simulink model "feedback_system"  (R2015a)
settings: Solver=ode45  StartTime=0.0  StopTime=t_stop  MaxStep=1e-4  MinStep=1e-5  RelTol=1e-3
undefined symbols (not defined in the file): delta_a, delta_y, rho, wy
libraries: cstblocks x2, simulink x1
settings Model: Creator=Berk Delibalta  LastModifiedBy=Berk Delibalta
settings SolverCC: InitialStep=1e-5

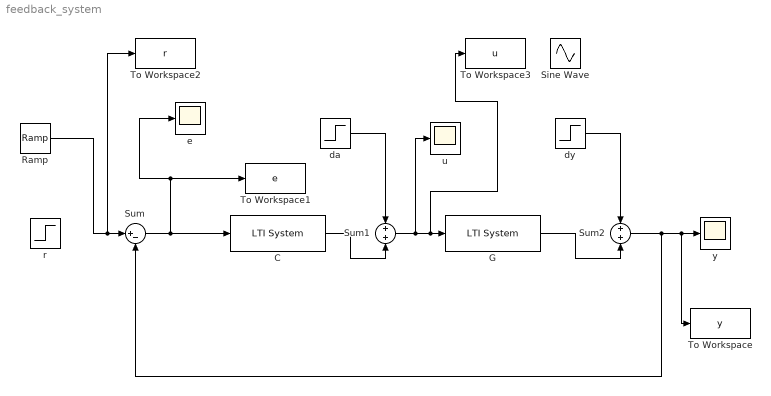
== system feedback_system ==
  C : cstblocks/LTI System  sys=C_ss  IC=[]
  G : cstblocks/LTI System  sys=G  IC=[]
  Ramp : simulink/Sources/Ramp  slope=rho  start=0  X0=0
  Sine Wave : Sin  Amplitude=delta_y  Bias=delta_y  Frequency=wy  SampleTime=0
  Sum : Sum  Inputs=|+-
  Sum1 : Sum
  Sum2 : Sum
  To Workspace : ToWorkspace  VariableName=y  SaveFormat=Timeseries  SampleTime=-1
  To Workspace1 : ToWorkspace  VariableName=e  SaveFormat=Timeseries  SampleTime=-1
  To Workspace2 : ToWorkspace  VariableName=r  SaveFormat=Timeseries  SampleTime=-1
  To Workspace3 : ToWorkspace  VariableName=u  SaveFormat=Timeseries  SampleTime=-1
  da : Step  Time=0  After=delta_a  SampleTime=0
  "dy " : Step  Time=0  After=delta_y  SampleTime=0
  e : Scope
      settings: SaveName=ScopeData2
  r : Step  Time=0  After=rho  SampleTime=0
  u : Scope
  y : Scope
  wires:
  Sum/1 -> To Workspace1/1, e/1, C/1
  Sum1/1 -> u/1, To Workspace3/1, G/1
  C/1 -> Sum1/2
  G/1 -> Sum2/2
  Sum2/1 -> To Workspace/1, y/1, Sum/2
  da/1 -> Sum1/1
  "dy "/1 -> Sum2/1
  Ramp/1 -> To Workspace2/1, Sum/1
